simulink model "miniprojekt1_sim"  (R2022b)
settings: Solver=VariableStepAuto  StartTime=0.0  StopTime=10.0  RelTol=1e-3
values from neighbouring files (symbols this model uses):
  cp = 1000    [m.m]    (also in miniprojekt.m)
  Cvp = cp*rop*Vp    (= 108000)    [m.m]    (also in miniprojekt.m = 1500)
  Cvw = cp*rop*Vw    (= 216000)    [m.m]    (also in miniprojekt.m = 3000)
  dfk = 0    [m.m]
  dTkz = 0    [m.m]    (also in miniprojekt.m)
  dTzew = 0    [m.m]    (also in miniprojekt.m = 2)
  fk = qkN/(cp*rop*Tkz)    (= 0.47619047619)    [m.m]
  K1 = (cp*fk*rop*(Tkz - Twew))/(5*Twew-4*Tzew-Tp)    (= 51.9480519481)    [m.m]    (also in miniprojekt.m = 275)
  K2 = (K1*(Twew-Tp))/(4*(Tp-Tzew))    (= 1.85528756957)    [m.m]    (also in miniprojekt.m = 60)
  Kp = (1/4) *K1    (= 12.987012987)    [m.m]    (also in miniprojekt.m = 900)
  rop = 1.2    [m.m]    (also in miniprojekt.m)
  Tkz = TkzN    (= 35)    [m.m]
  Tp = TpN    (= 15)    [m.m]    (also in skrypt1.m = (Qg + Kcw*(Twew - Tzew))/Kcp + Tzew)
  Twew = ( (Qg *(Kcwp+Kcp)) / ( (Kcw*Kcwp) + (Kcw * Kcp) + (Kcwp*Kcp) ))+ Tzew(i)    [lab1.m]    (also in m.m = 20; skrypt1.m = (Qg + Kcp*(Tp - Tzew))/Kcw + Tzew)
  Tzew = -20:5:30    [lab1.m]    (also in m.m = -20; skrypt1.m = -30:5:30)
settings Model: Creator=Lab320  LastModifiedBy=micha
settings SolverCC: AlgebraicLoopSolver=TrustRegion
settings DebuggingCC: UnconnectedInputMsg=warning  UnconnectedOutputMsg=warning  UnconnectedLineMsg=warning  SFMachineParentedDataDiag=warning
settings ModelReferenceCC: EnableRefExpFcnMdlSchedulingChecks=on
settings RTWCC: DLArmComputeVersion=19.05

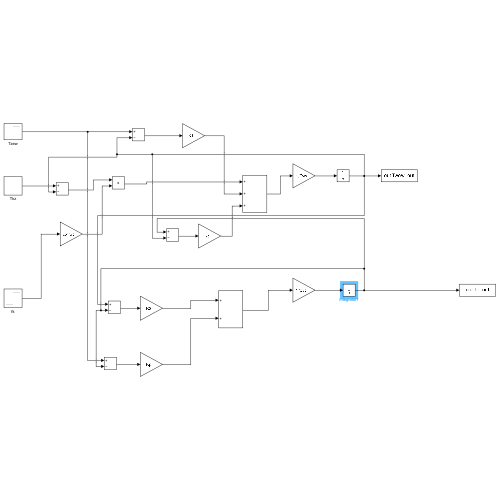
[thumbnail: Simulink's stored preview of the top-level diagram]
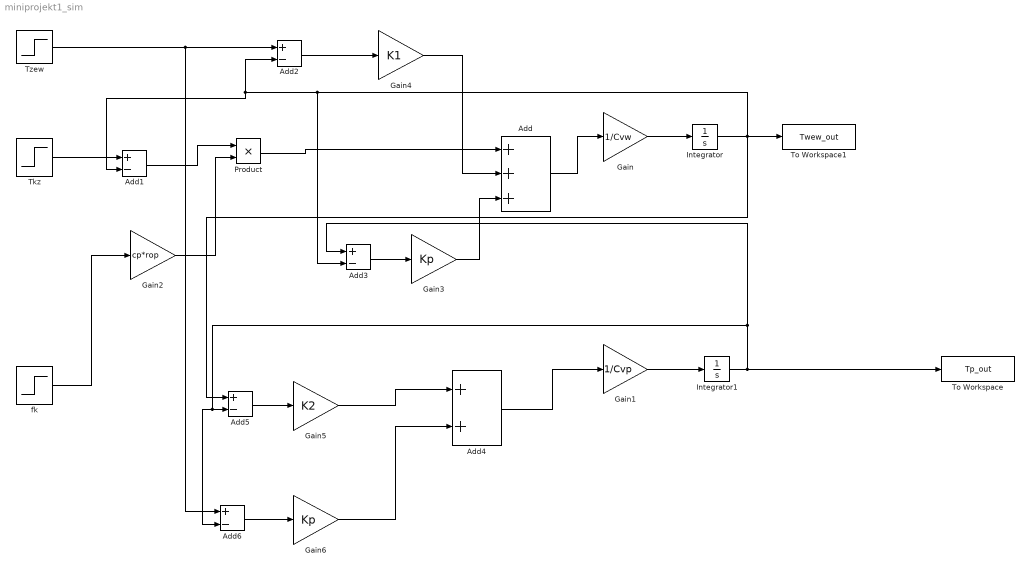
== system miniprojekt1_sim ==
  Add : Sum  Inputs=+++
  Add{1..3,5..6} (5 alike) : Sum  Inputs=+-
  Add4 : Sum
  Gain : Gain  Gain=1/Cvw
  Gain1 : Gain  Gain=1/Cvp
  Gain2 : Gain  Gain=cp*rop
  Gain3 : Gain  Gain=Kp
  Gain4 : Gain  Gain=K1
  Gain5 : Gain  Gain=K2
  Gain6 : Gain  Gain=Kp
  Integrator : Integrator  InitialCondition=Twew
  Integrator1 : Integrator  InitialCondition=Tp
  Product : Product
  Tkz : Step  Time=1000  Before=Tkz  After=Tkz+dTkz  SampleTime=0  ZeroCross=off
  To Workspace : ToWorkspace  VariableName=Tp_out  SampleTime=-1
  To Workspace1 : ToWorkspace  VariableName=Twew_out  SampleTime=-1
  Tzew : Step  Time=1000  Before=Tzew  After=Tzew + dTzew  SampleTime=0
  fk : Step  Time=1000  Before=fk  After=fk+dfk  SampleTime=0
  wires:
  Gain1/1 -> Integrator1/1
  Gain/1 -> Integrator/1
  Integrator1/1 -> Add5/2, Add6/2, Add3/1, To Workspace/1
  fk/1 -> Gain2/1
  Gain2/1 -> Product/2
  Product/1 -> Add/1
  Tkz/1 -> Add1/1
  Add1/1 -> Product/1
  Add2/1 -> Gain4/1
  Tzew/1 -> Add6/1, Add2/1
  Gain4/1 -> Add/2
  Gain3/1 -> Add/3
  Add3/1 -> Gain3/1
  Add/1 -> Gain/1
  Add4/1 -> Gain1/1
  Gain5/1 -> Add4/1
  Gain6/1 -> Add4/2
  Add5/1 -> Gain5/1
  Add6/1 -> Gain6/1
  Integrator/1 -> Add5/1, Add3/2, Add2/2, Add1/2, To Workspace1/1
